simulink model "andbot1dot2_ROScommand"  (R2015b)
settings: Solver=FixedStepAuto  StartTime=0.0  StopTime=inf  FixedStep=0.04  RelTol=1e-3
undefined symbols (not defined in the file or in its folder): Angular, Linear
libraries: robotlib x3, realtime_pacer_lib x2
settings Model: Creator=root  LastModifiedBy=root

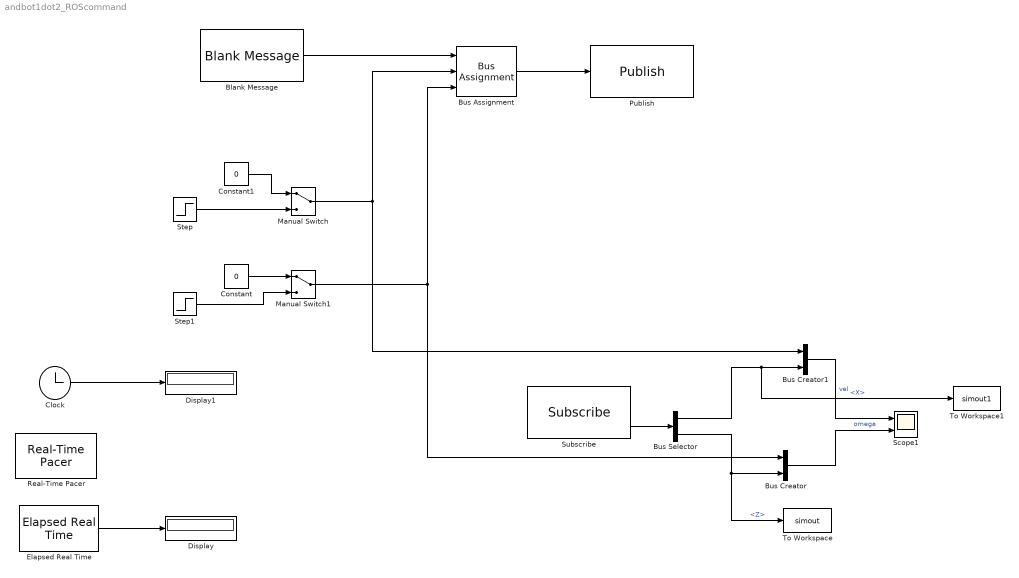
== system andbot1dot2_ROScommand ==
  Blank Message : robotlib/Blank Message  SourceLibraryInfo=This block requires Robotics System Toolbox  messageType=geometry_msgs/Twist  SampleTime=inf
  Bus Assignment : BusAssignment  AssignedSignals=Linear.X,Angular.Z
  Bus Creator : BusCreator  Inputs=2
  Bus Creator1 : BusCreator  Inputs=2
  Bus Selector : BusSelector  OutputSignals=Linear.X,Angular.Z
  Clock : Clock
  Constant : Constant  Value=0  OutDataTypeStr=double  SampleTime=-1
  Constant1 : Constant  Value=0  OutDataTypeStr=double  SampleTime=-1
  Display : Display
  Display1 : Display
  Elapsed Real Time : realtime_pacer_lib/Elapsed Real Time
  Manual Switch : ManualSwitch
  Manual Switch1 : ManualSwitch
  Publish : robotlib/Publish  SourceLibraryInfo=This block requires Robotics System Toolbox  topicSource=Select from ROS network  topic=/andbot1dot2/cmd_vel  messageType=geometry_msgs/Twist  messageQueueLength=1
  Real-Time Pacer : realtime_pacer_lib/Real-Time Pacer  simTimePerRealTime=1
  Scope1 : Scope  NumInputPorts=2
  Step : Step  Time=0  After=8
  Step1 : Step  Time=0
  Subscribe : robotlib/Subscribe  SourceLibraryInfo=This block requires Robotics System Toolbox  topicSource=Select from ROS network  topic=/andbot1dot2/feedback_Vel  messageType=geometry_msgs/Twist  sampleTime=-1  messageQueueLength=1
  To Workspace : ToWorkspace  VariableName=simout  SaveFormat=Timeseries  SampleTime=-1
  To Workspace1 : ToWorkspace  VariableName=simout1  SaveFormat=Timeseries  SampleTime=-1
  wires:
  Bus Assignment/1 -> Publish/1
  Blank Message/1 -> Bus Assignment/1
  Subscribe/2 -> Bus Selector/1
  Bus Selector/1 -> To Workspace1/1, Bus Creator1/2  "<X>"
  Bus Selector/2 -> Bus Creator/2, To Workspace/1  "<Z>"
  Manual Switch/1 -> Bus Creator1/1, Bus Assignment/2
  Constant1/1 -> Manual Switch/1
  Constant/1 -> Manual Switch1/1
  Manual Switch1/1 -> Bus Creator/1, Bus Assignment/3
  Bus Creator1/1 -> Scope1/1  "vel"
  Bus Creator/1 -> Scope1/2  "omega"
  Step/1 -> Manual Switch/2
  Step1/1 -> Manual Switch1/2
  Elapsed Real Time/1 -> Display/1
  Clock/1 -> Display1/1
